simulink model "mux"  (R2020a)
settings: Solver=VariableStepAuto  StartTime=0.0  StopTime=10.0  RelTol=1e-3
settings Model: Creator=11973  LastModifiedBy=11973

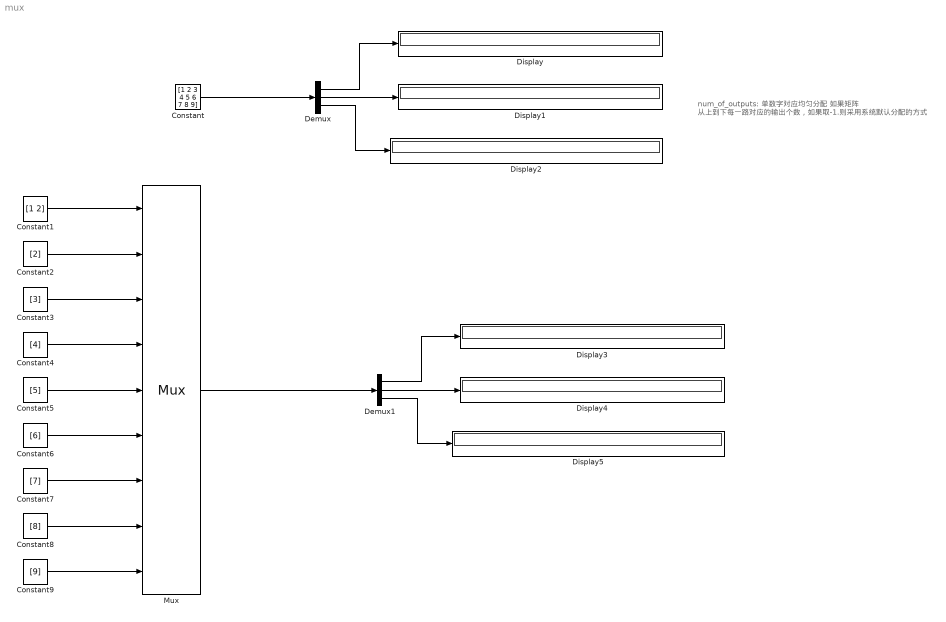
== system mux ==
  note: num_of_outputs: 单数字对应均匀分配
      | 如果矩阵 从上到下每一路对应的输出个数，如果取-1.则采用系统默认分配的方式
  Constant : Constant  Value=[1 2 3 4 5 6 7 8 9]  VectorParams1D=off
  Constant1 : Constant  Value=[1 2]  VectorParams1D=off
  Constant2 : Constant  Value=[2]  VectorParams1D=off
  Constant3 : Constant  Value=[3]  VectorParams1D=off
  Constant4 : Constant  Value=[4]  VectorParams1D=off
  Constant5 : Constant  Value=[5]  VectorParams1D=off
  Constant6 : Constant  Value=[6]  VectorParams1D=off
  Constant7 : Constant  Value=[7]  VectorParams1D=off
  Constant8 : Constant  Value=[8]  VectorParams1D=off
  Constant9 : Constant  Value=[9]  VectorParams1D=off
  Demux : Demux  Outputs=3
  Demux1 : Demux  Outputs=3
  Display{,1..5} (6 alike) : Display
  Mux : Mux  Inputs=9
  wires:
  Constant/1 -> Demux/1
  Demux/1 -> Display/1
  Demux/2 -> Display1/1
  Demux/3 -> Display2/1
  Demux1/3 -> Display5/1
  Demux1/2 -> Display4/1
  Demux1/1 -> Display3/1
  Mux/1 -> Demux1/1
  Constant2/1 -> Mux/2
  Constant3/1 -> Mux/3
  Constant4/1 -> Mux/4
  Constant5/1 -> Mux/5
  Constant6/1 -> Mux/6
  Constant7/1 -> Mux/7
  Constant8/1 -> Mux/8
  Constant9/1 -> Mux/9
  Constant1/1 -> Mux/1
